simulink model "Multi_Level_H_Bridge_5"  (R2014a)
settings: Solver=ode45  StartTime=0.0  StopTime=10.0  RelTol=1e-3
libraries: powerlib x14
settings Model: Creator=RAVINDERNATH YADAV  LastModifiedBy=RAVINDERNATH YADAV

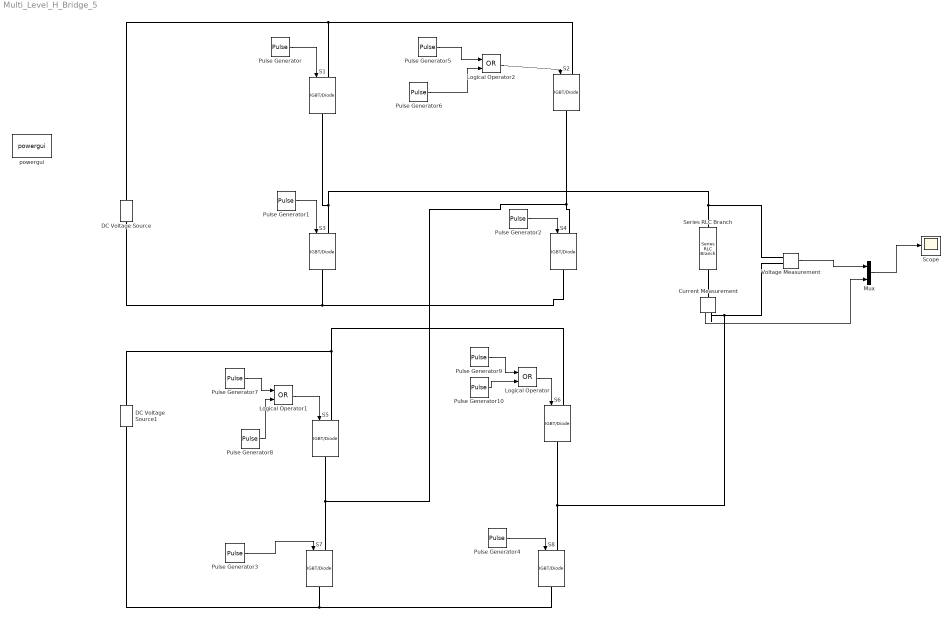
== system Multi_Level_H_Bridge_5 ==
  Current Measurement : powerlib/Measurements/Current Measurement  PhasorSimulation=off  OutputType=Complex  PSBequivalent=0
  DC Voltage Source : powerlib/Electrical Sources/DC Voltage Source  Amplitude=3  Measurements=None
  DC Voltage Source1 : powerlib/Electrical Sources/DC Voltage Source  Amplitude=3  Measurements=None
  Logical Operator : Logic  Operator=OR  AllPortsSameDT=off  OutDataTypeStr=boolean
  Logical Operator1 : Logic  Operator=OR  AllPortsSameDT=off  OutDataTypeStr=boolean
  Logical Operator2 : Logic  Operator=OR  AllPortsSameDT=off  OutDataTypeStr=boolean
  Mux : Mux  Inputs=2
  Pulse Generator : DiscretePulseGenerator  PulseType=Time based  Period=0.02  PulseWidth=(5/8)*100  PhaseDelay=(0.02/8)*0
  Pulse Generator1 : DiscretePulseGenerator  PulseType=Time based  Period=0.02  PulseWidth=(3/8)*100  PhaseDelay=(0.02/8)*5
  Pulse Generator10 : DiscretePulseGenerator  PulseType=Time based  Period=0.02  PulseWidth=(5/8)*100  PhaseDelay=(0.02/8)*3
  Pulse Generator2 : DiscretePulseGenerator  PulseType=Time based  Period=0.02  PulseWidth=(3/8)*100  PhaseDelay=(0.02/8)*1
  Pulse Generator3 : DiscretePulseGenerator  PulseType=Time based  Period=0.02  PulseWidth=(1/8)*100  PhaseDelay=(0.02/8)*6
  Pulse Generator4 : DiscretePulseGenerator  PulseType=Time based  Period=0.02  PulseWidth=(1/8)*100  PhaseDelay=(0.02/8)*2
  Pulse Generator5 : DiscretePulseGenerator  PulseType=Time based  Period=0.02  PulseWidth=(1/8)*100  PhaseDelay=(0.02/8)*0
  Pulse Generator6 : DiscretePulseGenerator  PulseType=Time based  Period=0.02  PulseWidth=(4/8)*100  PhaseDelay=(0.02/8)*4
  Pulse Generator7 : DiscretePulseGenerator  PulseType=Time based  Period=0.02  PulseWidth=(6/8)*100  PhaseDelay=(0.02/8)*0
  Pulse Generator8 : DiscretePulseGenerator  PulseType=Time based  Period=0.02  PulseWidth=(1/8)*100  PhaseDelay=(0.02/8)*7
  Pulse Generator9 : DiscretePulseGenerator  PulseType=Time based  Period=0.02  PulseWidth=(2/8)*100  PhaseDelay=(0.02/8)*0
  S{1..8} (8 alike) : powerlib/Power Electronics/IGBT//Diode  Ron=1e-3  Rs=1e5  Cs=inf  Measurements=off
  Scope : Scope
      settings: TimeRange=1
  Series RLC Branch : powerlib/Elements/Series RLC Branch  LConnTagsString=__new0  RConnTagsString=__new0  BranchType=R  Resistance=10  Inductance=1e-3  SetiL0=off  InitialCurrent=0  Capacitance=1e-6  Setx0=off  InitialVoltage=0  Measurements=None
  Voltage Measurement : powerlib/Measurements/Voltage Measurement  PhasorSimulation=off  OutputType=Complex  PSBequivalent=0
  powergui : powerlib/powergui  Priority=1  SimulationMode=Discrete  SolverType=Tustin  SampleTime=50e-6  frequency=60  SPID=off  DisableSnubberDevices=off  DisableRonSwitches=off  DisableVfSwitches=off  SwTol=0  Interpol=off  DisplayEquations=off  Ts=0  methode=off  frequencyindice=0  Pbase=100e6  ErrMax=1e-4  Iterations=50  UnitsV=kV  UnitsW=MW  FunctionMessages=off  echomessages=off  HookPort=off  EnableUseOfTLC=off  x0status=blocks  RestoreLinks=warning  ResistiveCurrentMeasurement=off  Frange=[0:2:500]  Ylog=off  Xlog=on  ShowGrid=off  save=off  variable=ZData  structure=logsout  ZoomFFT=off  StartTime=0.0  cycles=1  DisplayStyle=1  fundamental=50  FreqAxis=off  MaxFrequency=1000  frequencyindicesteady=1  RmsSteady=1  display=off
  wires:
  Voltage Measurement/1 -> Mux/1
  Pulse Generator/1 -> S1/1
  Pulse Generator5/1 -> Logical Operator2/1
  Pulse Generator6/1 -> Logical Operator2/2
  Logical Operator2/1 -> S2/1
  Pulse Generator1/1 -> S3/1
  Pulse Generator2/1 -> S4/1
  Pulse Generator7/1 -> Logical Operator1/1
  Pulse Generator8/1 -> Logical Operator1/2
  Logical Operator1/1 -> S5/1
  Pulse Generator9/1 -> Logical Operator/1
  Pulse Generator10/1 -> Logical Operator/2
  Logical Operator/1 -> S6/1
  Pulse Generator4/1 -> S8/1
  Pulse Generator3/1 -> S7/1
  Current Measurement/1 -> Mux/2
  Mux/1 -> Scope/1
  connections:
  S4/RConn1 -- S3/RConn1 -- DC Voltage Source/LConn1
  S3/LConn1 -- S1/RConn1 -- Series RLC Branch/LConn1 -- Voltage Measurement/LConn1
  S7/LConn1 -- S5/RConn1 -- S4/LConn1 -- S2/RConn1
  DC Voltage Source/RConn1 -- S1/LConn1 -- S2/LConn1
  S8/LConn1 -- S6/RConn1 -- Voltage Measurement/LConn2 -- Current Measurement/RConn1
  S5/LConn1 -- DC Voltage Source1/RConn1 -- S6/LConn1
  DC Voltage Source1/LConn1 -- S7/RConn1 -- S8/RConn1
  Series RLC Branch/RConn1 -- Current Measurement/LConn1
